simulink model "quadratic2006simulation"  (R2022b)
settings: Solver=VariableStepAuto  StartTime=0.0  StopTime=100  RelTol=1e-3
StartFcn:
  | run("scripts/quadratic2006parameters.m")
undefined symbols (not defined in the file): a, alpha1, alpha2, b, beta, c, DiscIntNeverNeededParam, f, g, gamma, h, kc, kn, kt, p, Vm
settings Model: Creator=kaganakar  LastModifiedBy=ASUS

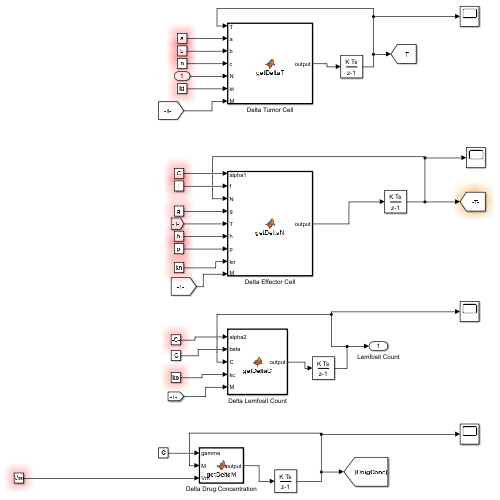
[thumbnail: Simulink's stored preview of the top-level diagram]
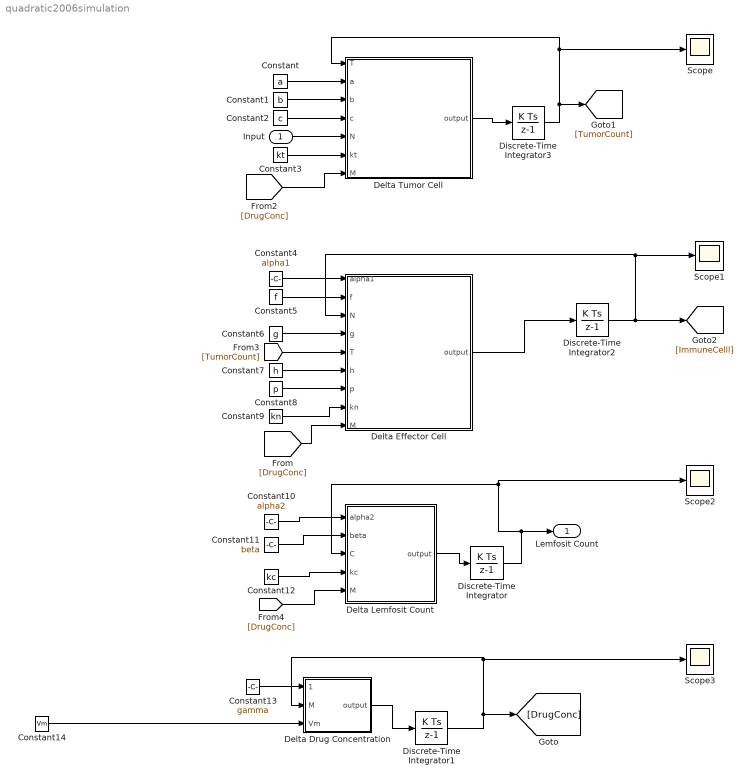
== system quadratic2006simulation ==
  Input : Inport
  Constant : Constant  Value=a
  Constant1 : Constant  Value=b
  Constant10 : Constant  Value=alpha2
  Constant11 : Constant  Value=beta
  Constant12 : Constant  Value=kc
  Constant13 : Constant  Value=gamma
  Constant14 : Constant  Value=Vm
  Constant2 : Constant  Value=c
  Constant3 : Constant  Value=kt
  Constant4 : Constant  Value=alpha1
  Constant5 : Constant  Value=f
  Constant6 : Constant  Value=g
  Constant7 : Constant  Value=h
  Constant8 : Constant  Value=p
  Constant9 : Constant  Value=kn
  Delta Drug Concentration : MATLAB Function  TreatAsAtomicUnit=on
  Delta Effector Cell : MATLAB Function  TreatAsAtomicUnit=on
  Delta Lemfosit Count : MATLAB Function  TreatAsAtomicUnit=on
  Delta Tumor Cell : MATLAB Function  TreatAsAtomicUnit=on
  Discrete-Time Integrator : DiscreteIntegrator  InitialCondition=6.25*10^10  ICPrevOutput=DiscIntNeverNeededParam  ICPrevScaledInput=DiscIntNeverNeededParam
  Discrete-Time Integrator1 : DiscreteIntegrator  ICPrevOutput=DiscIntNeverNeededParam  ICPrevScaledInput=DiscIntNeverNeededParam
  Discrete-Time Integrator2 : DiscreteIntegrator  InitialCondition=3*10^5  ICPrevOutput=DiscIntNeverNeededParam  ICPrevScaledInput=DiscIntNeverNeededParam
  Discrete-Time Integrator3 : DiscreteIntegrator  InitialCondition=10^7  ICPrevOutput=DiscIntNeverNeededParam  ICPrevScaledInput=DiscIntNeverNeededParam
  Scope{,1..3} (4 alike) : Scope
  Lemfosit Count : Outport
  wires:
  Delta Effector Cell/1(output) -> Discrete-Time Integrator2/1
  Discrete-Time Integrator2/1 -> Scope1/1, Delta Effector Cell/3(N), [ImmuneCelll]
  Delta Tumor Cell/1(output) -> Discrete-Time Integrator3/1
  Discrete-Time Integrator3/1 -> [TumorCount], Scope/1, Delta Tumor Cell/1(T)
  Input/1 -> Delta Tumor Cell/5(N)
  [TumorCount] -> Delta Effector Cell/5(T)
  Delta Lemfosit Count/1(output) -> Discrete-Time Integrator/1
  Discrete-Time Integrator/1 -> Scope2/1, Delta Lemfosit Count/3(C), Lemfosit Count/1
  Delta Drug Concentration/1(output) -> Discrete-Time Integrator1/1
  Discrete-Time Integrator1/1 -> Scope3/1, Delta Drug Concentration/2(M), [DrugConc]
  [DrugConc] -> Delta Lemfosit Count/5(M)
  [DrugConc] -> Delta Effector Cell/9(M)
  Constant/1 -> Delta Tumor Cell/2(a)
  Constant1/1 -> Delta Tumor Cell/3(b)
  Constant2/1 -> Delta Tumor Cell/4(c)
  Constant3/1 -> Delta Tumor Cell/6(kt)
  [DrugConc] -> Delta Tumor Cell/7(M)
  Constant5/1 -> Delta Effector Cell/2(f)
  Constant4/1 -> Delta Effector Cell/1(alpha1)
  Constant6/1 -> Delta Effector Cell/4(g)
  Constant7/1 -> Delta Effector Cell/6(h)
  Constant8/1 -> Delta Effector Cell/7(p)
  Constant9/1 -> Delta Effector Cell/8(kn)
  Constant10/1 -> Delta Lemfosit Count/1(alpha2)
  Constant11/1 -> Delta Lemfosit Count/2(beta)
  Constant12/1 -> Delta Lemfosit Count/4(kc)
  Constant13/1 -> Delta Drug Concentration/1(gamma)
  Constant14/1 -> Delta Drug Concentration/3(Vm)

== matlab function quadratic2006simulation/Delta Tumor Cell ==
  data: T input; a input; b input; c input; output output; N input; kt input; M input
function output = getDeltaT(T, a, b, c, N, kt, M)
    output = a*T*(1-b*T)-c*N*T - kt*M*T;
end

== matlab function quadratic2006simulation/Delta Effector Cell ==
  data: alpha1 input; f input; output output; N input; g input; T input; h input; p input; kn input; M input
function output = getDeltaN(alpha1,f,N,g,T,h,p,kn,M)
    output = alpha1-f*N+g*(T)/(h+T)*N - p*N*T - kn*M*N;
end

== matlab function quadratic2006simulation/Delta Lemfosit Count ==
  data: alpha2 input; beta input; output output; C input; kc input; M input
function output = getDeltaC(alpha2,beta,C,kc,M)
    output = alpha2 - beta*C - kc*M*C;
end

== matlab function quadratic2006simulation/Delta Drug Concentration ==
  data: gamma input; M input; output output; Vm input
function output = getDeltaM(gamma,M, Vm)
    output = -gamma*M + Vm;
end
